simulink model "position"  (R2022b)
settings: Solver=FixedStepAuto  StartTime=0.0  StopTime=inf  RelTol=1e-3  EnableMultiTasking=on
libraries: arduinolib x4, simulink x1
settings Model: ExtModeTrigDuration=2  Creator=MO.Tarek  LastModifiedBy=dell
settings SolverCC: AlgebraicLoopSolver=TrustRegion  AutoInsertRateTranBlk=on
settings OptimizationCC: EnhancedBackFolding=on  PassReuseOutputArgsAs=Individual arguments  MaxStackSize=64  OptimizeBlockOrder=speed  DifferentSizesBufferReuse=on  OptimizationCustomize=off  EfficientTunableParamExpr=on
settings DebuggingCC: ParameterTunabilityLossMsg=error  UnconnectedInputMsg=warning  UnconnectedOutputMsg=warning  UnconnectedLineMsg=warning  ArithmeticOperatorsInVariantConditions=warning
settings HardwareCC: ProdBitPerInt=16  ProdBitPerPointer=16  ProdBitPerSizeT=16  ProdBitPerPtrDiffT=16  ProdLargestAtomicFloat=None  ProdWordSize=8  ProdHWDeviceType=Atmel->AVR
settings ModelReferenceCC: EnableRefExpFcnMdlSchedulingChecks=on
settings SFSimCC: MATLABDynamicMemAlloc=off  CustomCodeUndefinedFunction=UseInterfaceOnly
settings RTWCC: Description=Embedded Coder  SystemTargetFile=ert.tlc  HardwareBoard=Arduino Uno  TLCOptions=-aInlineSetEventsForThisBaseRateFcn=TLC_FALSE -aSuppressMultiTaskScheduler=TLC_FALSE -aRateBasedStepFcn=1  TemplateMakefile=ert_default_tmf  GenerateReport=on  Toolchain=Arduino AVR  BuildConfiguration=Faster Runs  IncludeHyperlinkInReport=on  LaunchReport=on  GenerateTraceInfo=on  GenerateTraceReport=on  GenerateTraceReportSl=on  GenerateTraceReportSf=on  GenerateTraceReportEml=on
settings CodeAppCC: ForceParamTrailComments=on  IgnoreCustomStorageClasses=off  OperatorAnnotations=on  SimulinkDataObjDesc=on  SFDataObjDesc=on  InsertBlockDesc=on
settings ERTTargetCC: SupportContinuousTime=on  SupportVariableSizeSignals=on

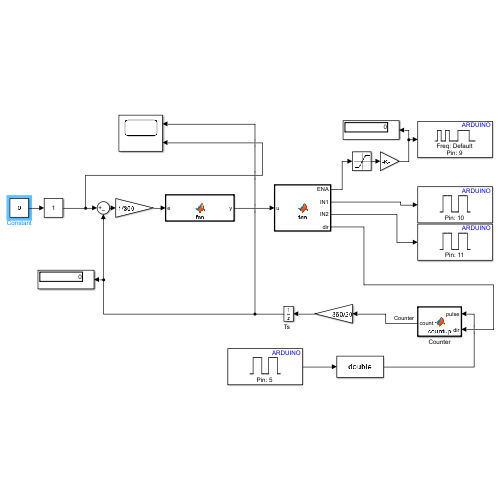
[thumbnail: Simulink's stored preview of the top-level diagram]
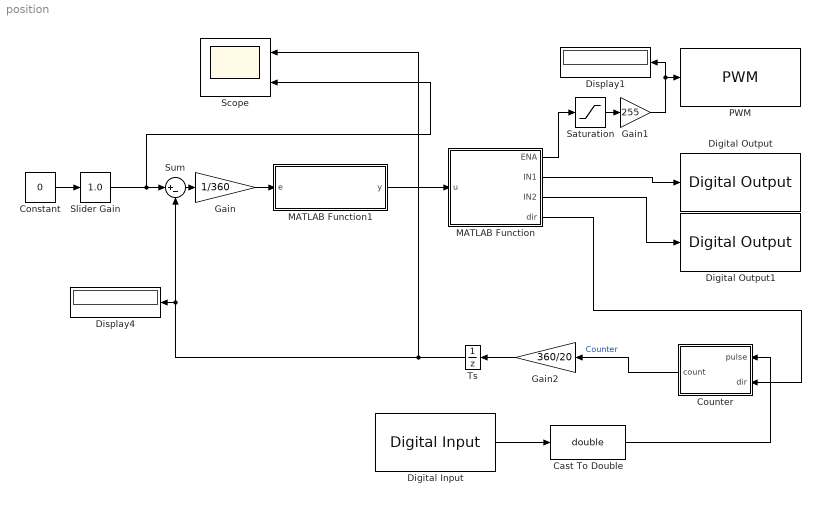
== system position ==
  Cast To Double : DataTypeConversion  OutDataTypeStr=double  SaturateOnIntegerOverflow=off  RndMeth=Floor
  Constant : Constant  Value=0  SampleTime=0.01
  Counter : MATLAB Function  TreatAsAtomicUnit=on  SystemSampleTime=0.01
  Digital Input : arduinolib/Digital Input  pinNumber=5  mode=Default  Direction=input  SampleTime=0.01  blockPlatform=arduino
  Digital Output : arduinolib/Digital Output  pinNumber=10  Direction=output  blockPlatform=arduino
  Digital Output1 : arduinolib/Digital Output  pinNumber=11  Direction=output  blockPlatform=arduino
  Display1 : Display
  Display4 : Display
  Gain : Gain  Gain=1/360
  Gain1 : Gain  Gain=255
  Gain2 : Gain  Gain=360/20
  MATLAB Function : MATLAB Function  TreatAsAtomicUnit=on  SystemSampleTime=0.01
  MATLAB Function1 : MATLAB Function  TreatAsAtomicUnit=on
  PWM : arduinolib/PWM  pinNumber=9  frequencyType=Default  desiredFrequency=490.2  achievableFrequency=490.2
  Saturation : Saturate  UpperLimit=1  LowerLimit=-1
  Scope : Scope  NumInputPorts=2
  Slider Gain : simulink/Math Operations/Slider Gain  gain=1.0  low=0  high=1
  Sum : Sum  Inputs=|+-
  "Ts  " : UnitDelay  SampleTime=0.01  HasFrameUpgradeWarning=on
  wires:
  Counter/1(count) -> Gain2/1  "Counter"
  "Ts  "/1 -> Scope/1, Display4/1, Sum/2
  MATLAB Function/1(ENA) -> Saturation/1
  Saturation/1 -> Gain1/1
  MATLAB Function/4(dir) -> Counter/2(dir)
  Gain1/1 -> Display1/1, PWM/1
  Constant/1 -> Slider Gain/1
  MATLAB Function/2(IN1) -> Digital Output/1
  Gain2/1 -> "Ts  "/1
  Sum/1 -> Gain/1
  Cast To Double/1 -> Counter/1(pulse)
  MATLAB Function/3(IN2) -> Digital Output1/1
  Digital Input/1 -> Cast To Double/1
  Gain/1 -> MATLAB Function1/1(e)
  MATLAB Function1/1(y) -> MATLAB Function/1(u)
  Slider Gain/1 -> Scope/2, Sum/1

== matlab function position/Counter ==
  settings: updateMethod=DISCRETE
  data: pulse input; count output; dir input
function count = countup(pulse,dir)
    persistent c p
    if isempty(c)
        c = 0;
        p = 0;
    end
    if (p == 0 && pulse == 1)
       c = c+dir; 
    end
    p = pulse;
    count = c ;
end

== matlab function position/MATLAB Function ==
  data: u input; ENA output; IN1 output; IN2 output; dir output
function [ENA,IN1,IN2,dir] = fcn(u)
ENA=abs(u);
if u<0
    IN1=1; IN2=0;
    dir = -1;
elseif u>0 
    IN1=0; IN2=1;
    dir = 1;
else
    IN1=0; IN2=0;
    dir=1;
end

== matlab function position/MATLAB Function1 ==
  data: e input; y output
function y = fcn(e)

y =e;
KP=2;
KI=0.8;
Io=1;
Ts=0.01;
eo=1;
In=Io+eo*Ts
PI=KP*e+KI*In
Io=In;
eo=e;


% 
% y =e;
% KP=1.5;
% KI=0.1;
% Io=1;
% Ts=0.01;
% eo=1;
% In=Io+eo*Ts
% PI=KP*e+KI*In
% Io=In;
% eo=e;
